simulink model "RL_based_microgrid"  (R2024b)
settings: Solver=VariableStepAuto  StartTime=0.0  StopTime=24  RelTol=1e-3
undefined symbols (not defined in the file): dspblkCoreblockFVToolHelper, gcbh, Ion, Lithium
libraries: spsParallelRLCBranchLib x7, spsSeriesRLCBranchLib x6, spsCurrentMeasurementLib x4, spsPWMGeneratorDCDCLib x4, spsVoltageMeasurementLib x4, spsUniversalBridgeLib x3, spsIGBTDiodeLib x2, spsDiodeLib x2, spsIGBTLib x2, spsBatteryLib x1, spsExcitationSystemLib x1, slpidlib x1
settings Model: Creator=purna  LastModifiedBy=purna

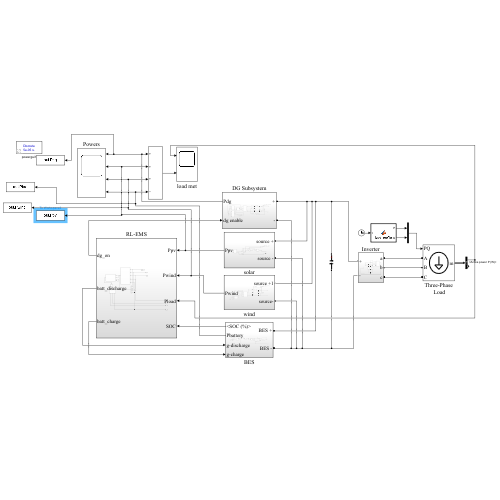
[thumbnail: Simulink's stored preview of the top-level diagram]
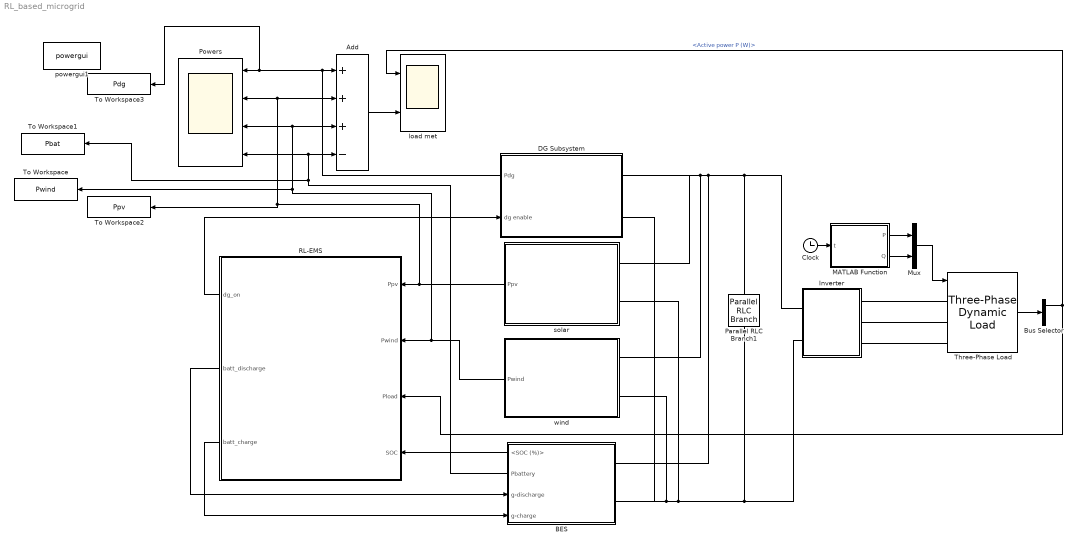
== system RL_based_microgrid ==
  Add : Sum  Inputs=+++-
  BES : Subsystem
      settings: PortSchema="{\"entries\":[{\"content\":{\"sides\":[{\"content\":{\"connectorIds\":[\"Out1\",\"Out2\",\"In1\",\"In2\"]},\"type\":\"ConnectorPlacement.EquallySpacedRectSide\",\"uuid\":\"4ddb1c12-991e-4618-8b5a-96153a6be9f9\"},{\"content\":{\"connectorIds\":[\"RConn1\",\"RConn2\"],\"side\":\"RIGHT\"},\"type\":\"ConnectorPlacement.EquallySpacedRectSide\",\"uuid\":\"57b35f38-742b-43df-b310-85bef7c22eb6\"},{\"content\":{\"side\":\"TOP\"},\"type\":\"ConnectorPlacement.EquallySpacedRectSide\",\"uuid\":\"e8572676-69f6-4b23-a9b1-c7da9405a7b0\"}]},\"type\":\"ConnectorPlacement.EquallySpacedConnector\",\"uuid\":\"66137947-70c4-42b3-9854-4ace8c633b7a\"}],\"packageUris\":[\"http://schema.mathworks.com/mf0/Connector/R2020b\"],\"version\":\"1.0\"}"
  Bus Selector : BusSelector  OutputSignals=Active power P (W),Reactive power Q (var)
  Clock : Clock
  DG Subsystem : Subsystem
      settings: PortSchema="{\"entries\":[{\"content\":{\"sides\":[{\"content\":{\"connectorIds\":[\"LConn1\",\"LConn2\"]},\"type\":\"ConnectorPlacement.EquallySpacedRectSide\",\"uuid\":\"0fe261cd-b61b-4009-ad1d-7ade665678a0\"},{\"content\":{\"connectorIds\":[\"Out1\",\"In1\"],\"side\":\"RIGHT\"},\"type\":\"ConnectorPlacement.EquallySpacedRectSide\",\"uuid\":\"7da4c722-b648-49c7-a33d-9b77a7c6f0e6\"},{\"content\":{\"side\":\"TOP\"},\"type\":\"ConnectorPlacement.EquallySpacedRectSide\",\"uuid\":\"52742111-5208-4731-a6b6-f9628022c544\"}]},\"type\":\"ConnectorPlacement.EquallySpacedConnector\",\"uuid\":\"59f2cf42-9f29-4a8f-af78-3ef44fb976f0\"}],\"packageUris\":[\"http://schema.mathworks.com/mf0/Connector/R2020b\"],\"version\":\"1.0\"}"
  Inverter : Subsystem
  MATLAB Function : MATLAB Function  TreatAsAtomicUnit=on
  Mux : Mux  Inputs=2
  Parallel RLC Branch1 : spsParallelRLCBranchLib/Parallel RLC Branch  LConnTagsString=a  RConnTagsString=__new0  BranchType=C  Resistance=1  Inductance=1e-3  SetiL0=off  InitialCurrent=0  Capacitance=2200e-6  Setx0=off  InitialVoltage=0  Measurements=Branch voltage
  Powers : Scope  NumInputPorts=4
  RL-EMS : Subsystem
  Three-Phase Load : spsThreePhaseDynamicLoadLib/Three-Phase Dynamic Load  NominalVoltage=[ 415 50 ]  ActiveReactivePowers=[12000 5810]  PositiveSequence=[0.994 -11.8]  ExternalControl=on  NpNq=[1.3 2]  TimeConstants="[0  0  0  0]"  MinimumVoltage=0.7  Tfilter=1e-4  LoadFlowParameters=[4,0,0,0,0]
      settings: LibrarySourceBlock=|
      | sps_lib/Passives/Three-Phase
      | Dynamic Load
  To Workspace : ToWorkspace  VariableName=Pwind  SampleTime=-1
  To Workspace1 : ToWorkspace  VariableName=Pbat  SampleTime=-1
  To Workspace2 : ToWorkspace  VariableName=Ppv  SampleTime=-1
  To Workspace3 : ToWorkspace  VariableName=Pdg  SampleTime=-1
  load met : Scope  NumInputPorts=2
  powergui1 : sps_lib/powergui  Priority=1  SimulationMode=Discrete  SampleTime=50e-6  frequency=60  Iterations=50  frequencyindice=0  Pbase=100e6  ErrMax=1e-4  UnitsV=kV  UnitsW=MW  buscounter=0  FunctionMessages=off  echomessages=off  EnableUseOfTLC=off  CurrentSourceSwitches=off  DisableSnubberDevices=off  DisableRonSwitches=off  DisableVfSwitches=off  DisplayEquations=off  AutomaticDiscreteSolvers=off  SolverType=Tustin/Backward Euler (TBE)  Interpol=off  ExternalGateDelay=off  methode=off  Ts=100  x0status=blocks  SPID=on  SwTol=0  HookPort=off  NonlinearTolerance=1e-4  nMaxIteration=100  ContinueOnMaxIteration=off  RestoreLinks=warning  ResistiveCurrentMeasurement=off  Frange=[0:2:500]  Ylog=off  Xlog=on  ShowGrid=off  save=off  variable=ZData  structure=0  ZoomFFT=off  StartTime=0.0  cycles=1  DisplayStyle=1  fundamental=60  FreqAxis=off  MaxFrequency=1000  frequencyindicesteady=1  RmsSteady=1  display=off
  solar : Subsystem
      settings: PortSchema="{\"entries\":[{\"content\":{\"sides\":[{\"content\":{\"connectorIds\":[\"Out1\"]},\"type\":\"ConnectorPlacement.EquallySpacedRectSide\",\"uuid\":\"4201751c-a9df-4880-bfb5-bb337a412f45\"},{\"content\":{\"connectorIds\":[\"RConn1\",\"RConn2\"],\"side\":\"RIGHT\"},\"type\":\"ConnectorPlacement.EquallySpacedRectSide\",\"uuid\":\"9e737d78-7a45-4b12-adbf-ff1ceeb3dd67\"},{\"content\":{\"side\":\"TOP\"},\"type\":\"ConnectorPlacement.EquallySpacedRectSide\",\"uuid\":\"1925966d-444e-49d2-aa13-9b6a49dc85cf\"}]},\"type\":\"ConnectorPlacement.EquallySpacedConnector\",\"uuid\":\"d7480a8d-0b50-46ad-a335-fcb334a83c63\"}],\"packageUris\":[\"http://schema.mathworks.com/mf0/Connector/R2020b\"],\"version\":\"1.0\"}"
  wind : Subsystem
      settings: PortSchema="{\"entries\":[{\"content\":{\"sides\":[{\"content\":{\"connectorIds\":[\"Out1\"]},\"type\":\"ConnectorPlacement.EquallySpacedRectSide\",\"uuid\":\"4201751c-a9df-4880-bfb5-bb337a412f45\"},{\"content\":{\"connectorIds\":[\"RConn1\",\"RConn2\"],\"side\":\"RIGHT\"},\"type\":\"ConnectorPlacement.EquallySpacedRectSide\",\"uuid\":\"9e737d78-7a45-4b12-adbf-ff1ceeb3dd67\"},{\"content\":{\"side\":\"TOP\"},\"type\":\"ConnectorPlacement.EquallySpacedRectSide\",\"uuid\":\"1925966d-444e-49d2-aa13-9b6a49dc85cf\"}]},\"type\":\"ConnectorPlacement.EquallySpacedConnector\",\"uuid\":\"d7480a8d-0b50-46ad-a335-fcb334a83c63\"}],\"packageUris\":[\"http://schema.mathworks.com/mf0/Connector/R2020b\"],\"version\":\"1.0\"}"
  wires:
  Mux/1 -> Three-Phase Load/1
  MATLAB Function/2(Q) -> Mux/2
  Clock/1 -> MATLAB Function/1(t)
  Three-Phase Load/1 -> Bus Selector/1
  MATLAB Function/1(P) -> Mux/1
  RL-EMS/3(batt_charge) -> BES/2(g-charge)
  RL-EMS/2(batt_discharge) -> BES/1(g-discharge)
  RL-EMS/1(dg_on) -> DG Subsystem/1(dg enable)
  solar/1(Ppv) -> Add/2, Powers/2, To Workspace2/1, RL-EMS/1(Ppv)
  wind/1(Pwind) -> RL-EMS/2(Pwind), Add/3, Powers/3, To Workspace/1
  BES/1(<SOC (%)>) -> RL-EMS/4(SOC)
  Bus Selector/1 -> RL-EMS/3(Pload), load met/1  "<Active power P (W)>"
  DG Subsystem/1(Pdg) -> To Workspace3/1, Powers/1, Add/1
  Add/1 -> load met/2
  BES/2(Pbattery) -> Add/4, Powers/4, To Workspace1/1
  connections:
  Inverter/RConn1 -- Parallel RLC Branch1/LConn1 -- BES/RConn1 -- wind/RConn1 -- DG Subsystem/LConn1 -- solar/RConn1
  solar/RConn2 -- wind/RConn2 -- DG Subsystem/LConn2 -- BES/RConn2 -- Parallel RLC Branch1/RConn1 -- Inverter/RConn2
  Three-Phase Load/LConn2 -- Inverter/LConn2
  Three-Phase Load/LConn3 -- Inverter/LConn3
  Three-Phase Load/LConn1 -- Inverter/LConn1

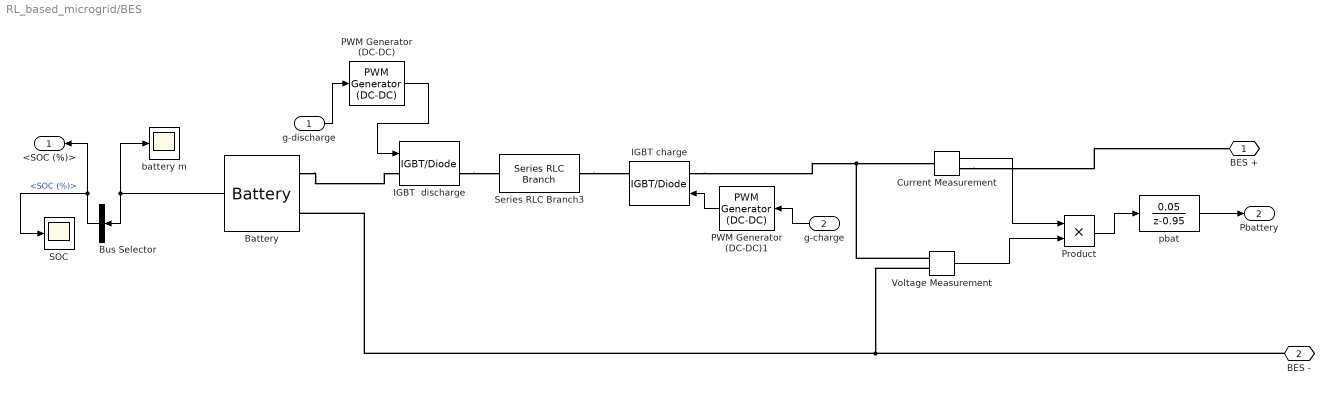
== system RL_based_microgrid/BES ==
  g-discharge : Inport
  g-charge : Inport  Port=2
  Battery : spsBatteryLib/Battery  BatType=Lithium-Ion  NomV=400  NomQ=50  SOC=60  Batt_Tr=0.5  PresetModel=on  MaxQ=50  MinV=300  FullV=465.5949  Dis_rate=21.7391  R=0.08  Normal_OP=45.2174  expZone="[432.1543      2.456522]"
  Bus Selector : BusSelector  OutputSignals=SOC (%)
  Current Measurement : spsCurrentMeasurementLib/Current Measurement  PhasorSimulation=off  OutputType=Complex  PSBequivalent=0
  IGBT  discharge : spsIGBTDiodeLib/IGBT//Diode  Ron=1e-3  Rs=1e5  Cs=inf  Measurements=on
  IGBT charge : spsIGBTDiodeLib/IGBT//Diode  Ron=1e-3  Rs=1e5  Cs=inf  Measurements=on
  PWM Generator (DC-DC) : spsPWMGeneratorDCDCLib/PWM Generator (DC-DC)  Fsw=50000  Ts=1e5
  PWM Generator (DC-DC)1 : spsPWMGeneratorDCDCLib/PWM Generator (DC-DC)  Fsw=50000  Ts=1e5
  Product : Product
  SOC : Scope
  Series RLC Branch3 : spsSeriesRLCBranchLib/Series RLC Branch  LConnTagsString=__new0  RConnTagsString=__new0  BranchType=L  Resistance=1  Inductance=2e-3  SetiL0=off  InitialCurrent=0  Capacitance=1e-6  Setx0=off  InitialVoltage=0  Measurements=None
  Voltage Measurement : spsVoltageMeasurementLib/Voltage Measurement  PhasorSimulation=off  OutputType=Complex  PSBequivalent=0
  battery m : Scope
  pbat : DiscreteTransferFcn  LoadFcn=dspblkCoreblockFVToolHelper(gcbh,'load');  Numerator=[0.05]  Denominator=[1 -0.95]
      settings: CopyFcn=dspblkCoreblockFVToolHelper(gcbh,'copy');  DeleteFcn=dspblkCoreblockFVToolHelper(gcbh,'close');  ModelCloseFcn=dspblkCoreblockFVToolHelper(gcbh,'close');  PreSaveFcn=dspblkCoreblockFVToolHelper(gcbh,'presave');  PostSaveFcn=dspblkCoreblockFVToolHelper(gcbh,'postsave');  CloseFcn=dspblkCoreblockFVToolHelper(gcbh,'close');
  BES + : PMIOPort  Side=Right
  BES - : PMIOPort  Port=2  Side=Right
  <SOC (%)> : Outport
  Pbattery : Outport  Port=2
  wires:
  Bus Selector/1 -> <SOC (%)>/1, SOC/1  "<SOC (%)>"
  Battery/1 -> Bus Selector/1, battery m/1
  g-discharge/1 -> PWM Generator (DC-DC)/1
  PWM Generator (DC-DC)/1 -> IGBT  discharge/1
  PWM Generator (DC-DC)1/1 -> IGBT charge/1
  g-charge/1 -> PWM Generator (DC-DC)1/1
  pbat/1 -> Pbattery/1
  Product/1 -> pbat/1
  Current Measurement/1 -> Product/1
  Voltage Measurement/1 -> Product/2
  connections:
  Series RLC Branch3/RConn1 -- IGBT charge/RConn1
  Battery/LConn1 -- IGBT  discharge/LConn1
  IGBT  discharge/RConn1 -- Series RLC Branch3/LConn1
  BES -/RConn1 -- Voltage Measurement/LConn2 -- Battery/LConn2
  IGBT charge/LConn1 -- Voltage Measurement/LConn1 -- Current Measurement/LConn1
  Current Measurement/RConn1 -- BES +/RConn1

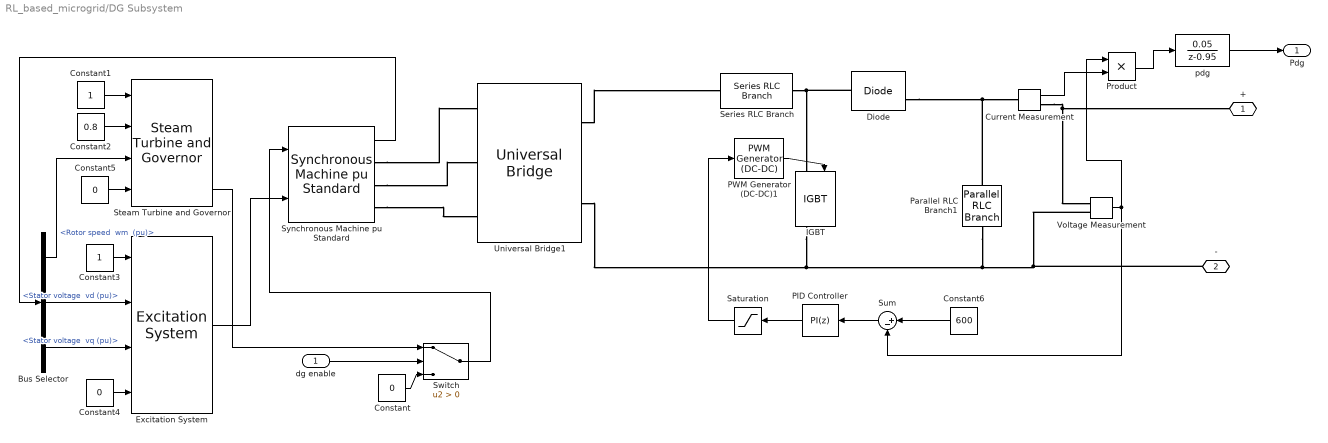
== system RL_based_microgrid/DG Subsystem ==
  dg enable : Inport
  Bus Selector : BusSelector  OutputSignals="Mechanical.Rotor speed  wm  (pu),dq0 components.Stator voltage  vd (pu),dq0 components.Stator voltage  vq (pu)"
  Constant : Constant  Value=0
  Constant1 : Constant
  Constant2 : Constant  Value=0.8
  Constant3 : Constant
  Constant4 : Constant  Value=0
  Constant5 : Constant  Value=0
  Constant6 : Constant  Value=600
  Current Measurement : spsCurrentMeasurementLib/Current Measurement  PhasorSimulation=off  OutputType=Complex  PSBequivalent=0
  Diode : spsDiodeLib/Diode  Ron=0.001  Lon=0  Vf=0.8  IC=0  UseSnubber=0  Rs=500  Cs=0  Measurements=on
  Excitation System : spsExcitationSystemLib/Excitation System  tr=20e-3  reg=[200 0.02]  exc=[ 1, 0.8 ]  tgr=[ 0, 0 ]  damp=[ 0.001, 0.1 ]  sat=[ 0, 0 ]  lim=[-5 5 0]  v0=[1.0 1.0]
  IGBT : spsIGBTLib/IGBT  Ron=0.001  Lon=0  Vf=1  Tf=1e-6  Tt=2e-6  IC=0  Rs=1e5  Cs=inf  Measurements=on
  PID Controller : slpidlib/PID Controller  Controller=PI  Form=Parallel  TimeDomain=Discrete-time  UseExternalTs=off  SampleTime=5e-6  IntegratorMethod=Forward Euler  FilterMethod=Forward Euler  ControllerParametersSource=internal  P=0.002  I=2  UseKiTs=off  D=0  UseExternalDerivativeSource=off  N=100  UseFilter=on  TunerSelectOption=Transfer Function Based (PID Tuner App)  InitialConditionSource=internal  InitialConditionForIntegrator=0  InitialConditionForFilter=0  DifferentiatorICPrevScaledInput=0  ExternalReset=none  TrackingMode=off  Kt=1  LimitOutput=on  SatLimitsSource=internal  UpperSaturationLimit=0.9  LowerSaturationLimit=0  LinearizeAsGain=on  AntiWindupMode=clamping  Kb=1  LimitIntegrator=off  UpperIntegratorSaturationLimit=inf  LowerIntegratorSaturationLimit=-inf  POutMin=[]  POutMax=[]  IOutMin=[]  IOutMax=[]  DOutMin=[]  DOutMax=[]  NOutMin=[]  NOutMax=[]  SumOutMin=[]  SumOutMax=[]  SaturationOutMin=[]  SaturationOutMax=[]  PParamMin=[]  PParamMax=[]  IParamMin=[]  IParamMax=[]  DParamMin=[]  DParamMax=[]  NParamMin=[]  NParamMax=[]  KbParamMin=[]  KbParamMax=[]  KtParamMin=[]  KtParamMax=[]  KbOutMin=[]  KbOutMax=[]  KtOutMin=[]  KtOutMax=[]  IntegratorOutMin=[]  IntegratorOutMax=[]  FilterOutMin=[]  FilterOutMax=[]  SumI1OutMin=[]  SumI1OutMax=[]  SumI2OutMin=[]  SumI2OutMax=[]  SumI3OutMin=[]  SumI3OutMax=[]  SumI4OutMin=[]  SumI4OutMax=[]  SumDOutMin=[]  SumDOutMax=[]  DifferentiatorOutMin=[]  DifferentiatorOutMax=[]  FilterDiffOutCoefMin=[]  FilterDiffOutCoefMax=[]  ReciprocalOutMin=[]  ReciprocalOutMax=[]  SumDenOutMin=[]  SumDenOutMax=[]  SumNumOutMin=[]  SumNumOutMax=[]  DivideOutMin=[]  DivideOutMax=[]  UdiffTsProdOutMin=[]  UdiffTsProdOutMax=[]  NTsProdOutMin=[]  NTsProdOutMax=[]  UintegralTsProdOutMin=[]  UintegralTsProdOutMax=[]  UngainTsProdOutMin=[]  UngainTsProdOutMax=[]  ClampingZeroOutDataTypeStr=Inherit: Inherit via back propagation  ClampingZeroOutMin=[]  ClampingZeroOutMax=[]  FilterDenConstantOutDataTypeStr=Inherit: Inherit via back propagation  FilterDenConstantOutMin=[]  FilterDenConstantOutMax=[]  PCopyOutDataTypeStr=Inherit: Inherit via back propagation  PCopyOutMin=[]  PCopyOutMax=[]  NCopyOutDataTypeStr=Inherit: Inherit via back propagation  NCopyOutMin=[]  NCopyOutMax=[]  IntegratorContinuousStateAttributes=''  IntegratorStateMustResolveToSignalObject=off  IntegratorRTWStateStorageClass=Auto  FilterContinuousStateAttributes=''  FilterStateMustResolveToSignalObject=off  FilterRTWStateStorageClass=Auto  ParallelPVariant=InternalParameters  IdealPVariant=Disabled  IVariant=InternalParameters  DVariant=Disabled  IntegratorVariant=Discrete  SatVariant=Enabled  AWVariant=DiscClampingParallel  PCopyVariant=Disabled  TRVariant=Disabled  FdbkBlocksVariant=Forward  IdealPFdbkVariant=Disabled  SatFdbkVariant=Disabled  DerivativeFilterVariant=Disabled  NVariant=Disabled  NCopyVariant=Disabled_SignalSpec  FilterICVariant=Disabled  IntegratorICVariant=InternalICs  ExternalResetVariant=Disabled  TRSumVariant=Passthrough  SumFdbkVariant=Disabled  SumVariant=Sum_PI  TsampFilterVariant=InternalTs  TsampNgainVariant=Passthrough  TsampIntegralVariant=Disabled_SignalSpec  ExternalSaturationOutDataTypeStr=Inherit: Same as second input  DerivativeSourceVariant=Disabled  PreIntVariant=InternalPreInt
  PWM Generator (DC-DC)1 : spsPWMGeneratorDCDCLib/PWM Generator (DC-DC)  Fsw=10000  Ts=0
  Parallel RLC Branch1 : spsParallelRLCBranchLib/Parallel RLC Branch  LConnTagsString=a  RConnTagsString=__new0  BranchType=C  Resistance=1  Inductance=1e-3  SetiL0=off  InitialCurrent=0  Capacitance=2200e-6  Setx0=off  InitialVoltage=0  Measurements=None
  Product : Product
  Saturation : Saturate  UpperLimit=0.9  LowerLimit=0.02
  Series RLC Branch : spsSeriesRLCBranchLib/Series RLC Branch  LConnTagsString=__new0  RConnTagsString=__new0  BranchType=L  Resistance=1  Inductance=1e-3  SetiL0=off  InitialCurrent=0  Capacitance=1e-6  Setx0=off  InitialVoltage=0  Measurements=None
  Steam Turbine and Governor : spsSteamTurbineandGovernorLib/Steam Turbine and Governor  gentype=Tandem-compound (multi-mass)  reg1="[ 1  0.05    0 ]"  reg2="[ 0.001  0.15 ]"  reg3="[ -0.1  0.1  0  4.496]"  N=3600  turb1="[ 0  10   3.3   0.5   ]"  turb2="[ 0.5   0.5   0  0 ]"  HA="[  1.5498   0.24894  0  0 ]"  KA="[  83.47  42.702  0  0 ]"  DA="[  0.3104  0.05  0  0 ]*8"  ini1=250.35/555  ini2=[2.7247e-008,-120.13]
  Sum : Sum  Inputs=|+-
  Switch : Switch  Criteria=u2 > Threshold  SaturateOnIntegerOverflow=off  InputSameDT=off
  Synchronous Machine pu Standard : spsSynchronousMachinepuStandardLib/Synchronous Machine pu Standard  PresetModel=No  MechanicalLoad=Mechanical power Pm  ShowDetailedParameters=on  RotorType=Salient-pole  Units=per unit standard parameters  MeasurementBus=off  NominalParameters="[ 50e3   415   50   2 ]"  Reactances1=[ 1.81, 0.3, 0.23, 1.76, 0.65, 0.25, 0.15 ]  Reactances2=[2.24 0.17 0.12 1.02 0.13 0.08]  dAxisTimeConstants=Short-circuit  qAxisTimeConstants=Short-circuit  TimeConstants1="[ 4.4849  0.0681  0.1  ]"  TimeConstants2=[ 8.0, 0.03, 1.0, 0.07 ]  TimeConstants3="[  4.49  0.0681  0.0513  ]"  TimeConstants4=[ 8.0, 0.03, 0.3371, 0.0295 ]  TimeConstants5=[ 1.01, 0.053, 0.1 ]  TimeConstants6=[ 1.3201, 0.023, 1.0, 0.07 ]  TimeConstants7=[0.012 0.003 0.003]  TimeConstants8=[ 1.3201, 0.0231, 0.3371, 0.0295 ]  StatorResistance=0.037875  Mechanical=[0.1028 0.02056 2]  PolePairs=20  InitialConditions="[ 0  0  0  0  0  0  0  0  1 ]"  SetSaturation=off  Saturation=[0.6404,0.7127,0.8441,0.9214,0.9956,1.082,1.19,1.316,1.457;0.7,0.7698,0.8872,0.9466,0.9969,1.046,1.1,1.151,1.201]  LoadFlowParameters=[1,0,0,0,0]  TsPowergui=0  TsBlock=5e-05  IterativeModel=Trapezoidal non iterative  IterativeDiscreteModel=Trapezoidal non iterative  BusType=swing  Pref=20000  Qref=0  Qmin=-15000  Qmax=15000  PLF=0  QLF=0
  Universal Bridge1 : spsUniversalBridgeLib/Universal Bridge  Arms=3  SnubberResistance=1e5  SnubberCapacitance=inf  Device=Diodes  Ron=1e-3  Lon=0  ForwardVoltages="[  0  0  ]"  ForwardVoltage=0  GTOparameters=[ 10e-6 , 20e-6 ]  IGBTparameters=[ 1e-6 , 2e-6 ]  Measurements=None  Measurements_2=None  converterType=Rectifier
  Voltage Measurement : spsVoltageMeasurementLib/Voltage Measurement  PhasorSimulation=off  OutputType=Complex  PSBequivalent=0
  pdg : DiscreteTransferFcn  LoadFcn=dspblkCoreblockFVToolHelper(gcbh,'load');  Numerator=[0.05]  Denominator=[1 -0.95]
      settings: CopyFcn=dspblkCoreblockFVToolHelper(gcbh,'copy');  DeleteFcn=dspblkCoreblockFVToolHelper(gcbh,'close');  ModelCloseFcn=dspblkCoreblockFVToolHelper(gcbh,'close');  PreSaveFcn=dspblkCoreblockFVToolHelper(gcbh,'presave');  PostSaveFcn=dspblkCoreblockFVToolHelper(gcbh,'postsave');  CloseFcn=dspblkCoreblockFVToolHelper(gcbh,'close');
  + : PMIOPort  Side=Left
  - : PMIOPort  Port=2  Side=Left
  Pdg : Outport
  wires:
  Constant3/1 -> Excitation System/1
  Bus Selector/3 -> Excitation System/3  "<Stator voltage  vq (pu)>"
  Constant4/1 -> Excitation System/4
  Bus Selector/1 -> Steam Turbine and Governor/3  "<Rotor speed  wm  (pu)>"
  Constant2/1 -> Steam Turbine and Governor/2
  Bus Selector/2 -> Excitation System/2  "<Stator voltage  vd (pu)>"
  Constant1/1 -> Steam Turbine and Governor/1
  Constant5/1 -> Steam Turbine and Governor/4
  Excitation System/1 -> Synchronous Machine pu Standard/2
  Synchronous Machine pu Standard/1 -> Bus Selector/1
  Constant/1 -> Switch/3
  dg enable/1 -> Switch/2
  Product/1 -> pdg/1
  Current Measurement/1 -> Product/2
  pdg/1 -> Pdg/1
  Steam Turbine and Governor/4 -> Switch/1
  Switch/1 -> Synchronous Machine pu Standard/1
  PWM Generator (DC-DC)1/1 -> IGBT/1
  Voltage Measurement/1 -> Sum/2, Product/1
  Sum/1 -> PID Controller/1
  Saturation/1 -> PWM Generator (DC-DC)1/1
  PID Controller/1 -> Saturation/1
  Constant6/1 -> Sum/1
  connections:
  Synchronous Machine pu Standard/RConn3 -- Universal Bridge1/LConn3
  Synchronous Machine pu Standard/RConn1 -- Universal Bridge1/LConn1
  Synchronous Machine pu Standard/RConn2 -- Universal Bridge1/LConn2
  Parallel RLC Branch1/LConn1 -- Diode/RConn1 -- Current Measurement/LConn1
  IGBT/RConn1 -- Universal Bridge1/RConn2 -- Parallel RLC Branch1/RConn1 -- Voltage Measurement/LConn2 -- -/RConn1
  Current Measurement/RConn1 -- +/RConn1 -- Voltage Measurement/LConn1
  Series RLC Branch/RConn1 -- Diode/LConn1 -- IGBT/LConn1
  Universal Bridge1/RConn1 -- Series RLC Branch/LConn1

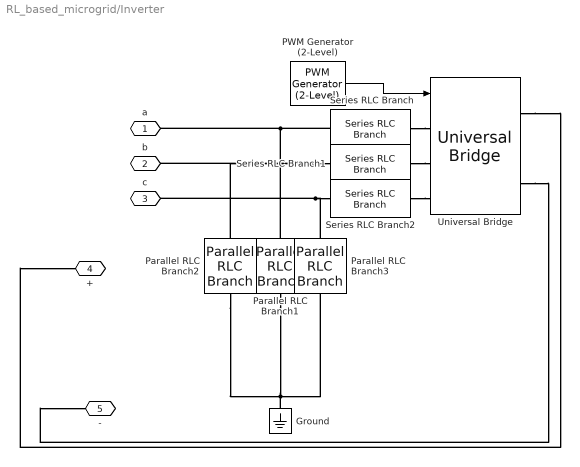
== system RL_based_microgrid/Inverter ==
  Ground : spsGroundLib/Ground  LConnTagsString=a
  PWM Generator (2-Level) : spsPWMGenerator2LevelLib/PWM Generator (2-Level)  ModulatorType=Three-phase bridge (6 pulses)  ModulatorMode=Unsynchronized  Fc=5000  Pc=0  nF=27  MinMax="[ -1  1 ]"  SamplingTechnique=Natural  ModulatingSignals=on  m=0.8  Freq=50  Phase=0  Ts=0  ShowCarrierOutport=off
  Parallel RLC Branch1 : spsParallelRLCBranchLib/Parallel RLC Branch  LConnTagsString=a  RConnTagsString=__new0  BranchType=C  Resistance=1  Inductance=1e-3  SetiL0=off  InitialCurrent=0  Capacitance=20e-6  Setx0=off  InitialVoltage=0  Measurements=None
  Parallel RLC Branch2 : spsParallelRLCBranchLib/Parallel RLC Branch  LConnTagsString=a  RConnTagsString=__new0  BranchType=C  Resistance=1  Inductance=1e-3  SetiL0=off  InitialCurrent=0  Capacitance=20e-6  Setx0=off  InitialVoltage=0  Measurements=None
  Parallel RLC Branch3 : spsParallelRLCBranchLib/Parallel RLC Branch  LConnTagsString=a  RConnTagsString=__new0  BranchType=C  Resistance=1  Inductance=1e-3  SetiL0=off  InitialCurrent=0  Capacitance=20e-6  Setx0=off  InitialVoltage=0  Measurements=None
  Series RLC Branch : spsSeriesRLCBranchLib/Series RLC Branch  LConnTagsString=__new0  RConnTagsString=__new0  BranchType=L  Resistance=1  Inductance=2e-3  SetiL0=off  InitialCurrent=0  Capacitance=1e-6  Setx0=off  InitialVoltage=0  Measurements=None
  Series RLC Branch1 : spsSeriesRLCBranchLib/Series RLC Branch  LConnTagsString=__new0  RConnTagsString=__new0  BranchType=L  Resistance=1  Inductance=2e-3  SetiL0=off  InitialCurrent=0  Capacitance=1e-6  Setx0=off  InitialVoltage=0  Measurements=None
  Series RLC Branch2 : spsSeriesRLCBranchLib/Series RLC Branch  LConnTagsString=__new0  RConnTagsString=__new0  BranchType=L  Resistance=1  Inductance=2e-3  SetiL0=off  InitialCurrent=0  Capacitance=1e-6  Setx0=off  InitialVoltage=0  Measurements=None
  Universal Bridge : spsUniversalBridgeLib/Universal Bridge  Arms=3  SnubberResistance=1e5  SnubberCapacitance=inf  Device=IGBT / Diodes  Ron=1e-3  Lon=0  ForwardVoltages="[  0  0  ]"  ForwardVoltage=0  GTOparameters=[ 10e-6 , 20e-6 ]  IGBTparameters=[ 1e-6 , 2e-6 ]  Measurements=None  Measurements_2=None  converterType=Rectifier
  a : PMIOPort  Side=Left
  b : PMIOPort  Port=2  Side=Left
  c : PMIOPort  Port=3  Side=Left
  + : PMIOPort  Port=4  Side=Right
  - : PMIOPort  Port=5  Side=Right
  wires:
  PWM Generator (2-Level)/1 -> Universal Bridge/1
  connections:
  Parallel RLC Branch2/RConn1 -- Ground/LConn1 -- Parallel RLC Branch1/RConn1 -- Parallel RLC Branch3/RConn1
  Series RLC Branch/RConn1 -- Universal Bridge/LConn1
  Series RLC Branch1/RConn1 -- Universal Bridge/LConn2
  Series RLC Branch2/RConn1 -- Universal Bridge/LConn3
  Universal Bridge/RConn2 -- -/RConn1
  Parallel RLC Branch3/LConn1 -- c/RConn1 -- Series RLC Branch2/LConn1
  Series RLC Branch/LConn1 -- Parallel RLC Branch1/LConn1 -- a/RConn1
  Universal Bridge/RConn1 -- +/RConn1
  Series RLC Branch1/LConn1 -- b/RConn1 -- Parallel RLC Branch2/LConn1

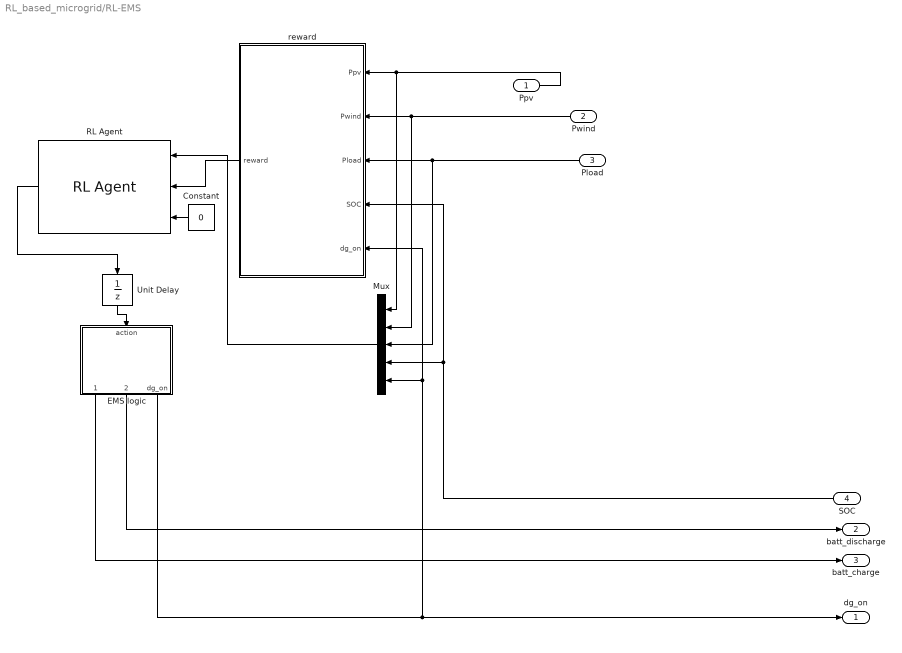
== system RL_based_microgrid/RL-EMS ==
  Ppv : Inport
  Pwind : Inport  Port=2
  Pload : Inport  Port=3
  SOC : Inport  Port=4
  Constant : Constant  Value=0
  EMS logic : MATLAB Function  TreatAsAtomicUnit=on
  Mux : Mux  Inputs=5
  RL Agent : rllib/RL Agent  Agent=agentObj  ExternalActionAsInput=off  ProvideLastAction=off  ProvideCumRwd=off  TreatAsDirectFeedthrough=on  UseStrictObservationDataTypes=off
  Unit Delay : UnitDelay  InitialCondition=2  SampleTime=-1  HasFrameUpgradeWarning=on
  reward : MATLAB Function  TreatAsAtomicUnit=on
  dg_on : Outport
  batt_discharge : Outport  Port=2
  batt_charge : Outport  Port=3
  wires:
  Constant/1 -> RL Agent/3
  SOC/1 -> reward/4(SOC), Mux/4
  Pload/1 -> Mux/3, reward/3(Pload)
  EMS logic/3(dg_on) -> dg_on/1, reward/5(dg_on), Mux/5
  Pwind/1 -> Mux/2, reward/2(Pwind)
  Ppv/1 -> Mux/1, reward/1(Ppv)
  Mux/1 -> RL Agent/1
  RL Agent/1 -> Unit Delay/1
  reward/1(reward) -> RL Agent/2
  EMS logic/1(batt_charge) -> batt_charge/1
  EMS logic/2(batt_discharge) -> batt_discharge/1
  Unit Delay/1 -> EMS logic/1(action)

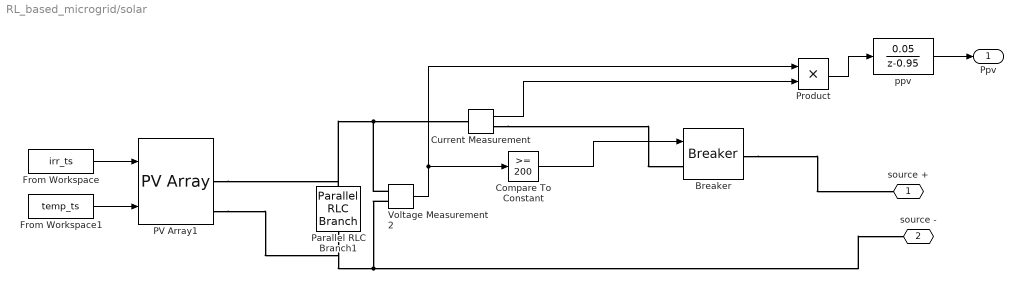
== system RL_based_microgrid/solar ==
  Breaker : spsBreakerLib/Breaker  InitialState=0  SwitchingTimes="[1/60  5/60]"  External=on  BreakerResistance=0.01  SnubberResistance=1e6  SnubberCapacitance=inf  Measurements=None  MoreParameters=on  NoBreakLoop=off
  Compare To Constant : simulink/Logic and Bit Operations/Compare To Constant  relop=>=  const=200  OutDataTypeStr=boolean
  Current Measurement : spsCurrentMeasurementLib/Current Measurement  PhasorSimulation=off  OutputType=Complex  PSBequivalent=0
  From Workspace : FromWorkspace  VariableName=irr_ts  SampleTime=0.01
  From Workspace1 : FromWorkspace  VariableName=temp_ts  SampleTime=0.01
  PV Array1 : spsPVArrayLib/PV Array  Npar=4  Nser=20  PlotType=array @ 1000 W/m2 & specified temperatures  S_vec="[ 1000  500  100 ]"  Temp_C_vec="[ 25 45  ]"  ModuleName=User-defined  PlotWhenSelected=off  Pm=324  Ncell=60  Voc=45  Isc=9.2  Vm=36  Im=9  beta_Voc_pc=-0.36099  alpha_Isc_pc=0.102  beta_Voc=-0.16245  alpha_Isc=0.009384  IL=9.4197  I0=3.4412e-10  nI=1.2147  Rsh=3652.5591  Rs=0.39728  RobustModel=off  RobustCellTemperature=313.3991  BAL=on  Tc=1e-6  Tfilter=5e-5
  Parallel RLC Branch1 : spsParallelRLCBranchLib/Parallel RLC Branch  LConnTagsString=a  RConnTagsString=__new0  BranchType=C  Resistance=1  Inductance=1e-3  SetiL0=off  InitialCurrent=0  Capacitance=2200e-6  Setx0=off  InitialVoltage=0  Measurements=None
  Product : Product
  Voltage Measurement2 : spsVoltageMeasurementLib/Voltage Measurement  PhasorSimulation=off  OutputType=Complex  PSBequivalent=0
  ppv : DiscreteTransferFcn  LoadFcn=dspblkCoreblockFVToolHelper(gcbh,'load');  Numerator=[0.05]  Denominator=[1 -0.95]
      settings: CopyFcn=dspblkCoreblockFVToolHelper(gcbh,'copy');  DeleteFcn=dspblkCoreblockFVToolHelper(gcbh,'close');  ModelCloseFcn=dspblkCoreblockFVToolHelper(gcbh,'close');  PreSaveFcn=dspblkCoreblockFVToolHelper(gcbh,'presave');  PostSaveFcn=dspblkCoreblockFVToolHelper(gcbh,'postsave');  CloseFcn=dspblkCoreblockFVToolHelper(gcbh,'close');
  source + : PMIOPort  Side=Right
  source - : PMIOPort  Port=2  Side=Right
  Ppv : Outport
  wires:
  From Workspace/1 -> PV Array1/1
  From Workspace1/1 -> PV Array1/2
  Current Measurement/1 -> Product/2
  Product/1 -> ppv/1
  Voltage Measurement2/1 -> Product/1, Compare To Constant/1
  ppv/1 -> Ppv/1
  Compare To Constant/1 -> Breaker/1
  connections:
  Voltage Measurement2/LConn1 -- PV Array1/RConn1 -- Parallel RLC Branch1/LConn1 -- Current Measurement/LConn1
  Voltage Measurement2/LConn2 -- Parallel RLC Branch1/RConn1 -- PV Array1/RConn2 -- source -/RConn1
  Current Measurement/RConn1 -- Breaker/LConn1
  Breaker/RConn1 -- source +/RConn1

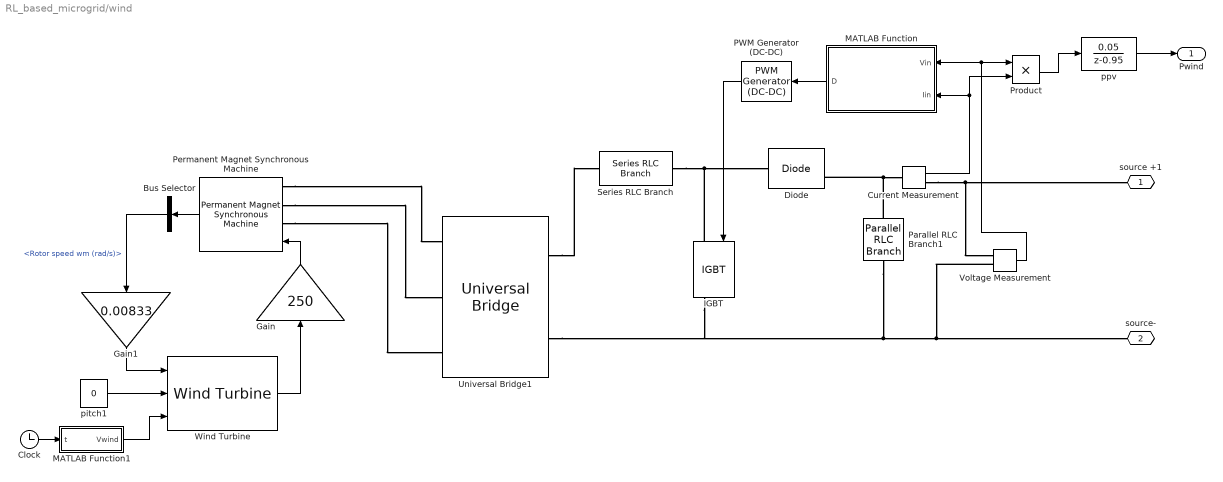
== system RL_based_microgrid/wind ==
  Bus Selector : BusSelector  OutputSignals=Rotor speed wm (rad/s)
  Clock : Clock
  Current Measurement : spsCurrentMeasurementLib/Current Measurement  PhasorSimulation=off  OutputType=Complex  PSBequivalent=0
  Diode : spsDiodeLib/Diode  Ron=0.001  Lon=0  Vf=0.8  IC=0  UseSnubber=0  Rs=500  Cs=0  Measurements=on
  Gain : Gain  Gain=250
  Gain1 : Gain  Gain=0.00833
  IGBT : spsIGBTLib/IGBT  Ron=0.001  Lon=0  Vf=1  Tf=1e-6  Tt=2e-6  IC=0  Rs=1e5  Cs=inf  Measurements=on
  MATLAB Function : MATLAB Function  TreatAsAtomicUnit=on
  MATLAB Function1 : MATLAB Function  TreatAsAtomicUnit=on
  PWM Generator (DC-DC) : spsPWMGeneratorDCDCLib/PWM Generator (DC-DC)  Fsw=10000  Ts=0
  Parallel RLC Branch1 : spsParallelRLCBranchLib/Parallel RLC Branch  LConnTagsString=a  RConnTagsString=__new0  BranchType=C  Resistance=1  Inductance=1e-3  SetiL0=off  InitialCurrent=0  Capacitance=1100e-6  Setx0=off  InitialVoltage=0  Measurements=Branch voltage
  Permanent Magnet Synchronous Machine : spsPermanentMagnetSynchronousMachineLib/Permanent Magnet Synchronous Machine  NbPhases=3  FluxDistribution=Sinusoidal  RotorType=Round  MechanicalLoad=Torque Tm  PresetModel=No  ShowDetailedParameters=on  MeasurementBus=off  Resistance=0.425  Inductance=8.5e-3  dqInductances=[8.5e-3,8.5e-3]  La=0.0085  MachineConstant=Flux linkage established by magnets (V.s)  Flux=0.433  VoltageCst=314.15  TorqueCst=2.598  Flat=120  Mechanical=[0.02 0.001 4 0]  PolePairs=4  InitialConditions=[0,0, 0,0]  InitialConditions5ph=[0 0 0 0 0 0]  RefAngle=90 degrees behind phase A axis (modified Park)  IterativeDiscreteModel=Trapezoidal non iterative  TsBlock=-1  TsPowergui=0
  Product : Product
  Series RLC Branch : spsSeriesRLCBranchLib/Series RLC Branch  LConnTagsString=__new0  RConnTagsString=__new0  BranchType=L  Resistance=1  Inductance=1e-3  SetiL0=off  InitialCurrent=0  Capacitance=1e-6  Setx0=off  InitialVoltage=0  Measurements=None
  Universal Bridge1 : spsUniversalBridgeLib/Universal Bridge  Arms=3  SnubberResistance=1e5  SnubberCapacitance=inf  Device=Diodes  Ron=1e-3  Lon=0  ForwardVoltages="[  0  0  ]"  ForwardVoltage=0  GTOparameters=[ 10e-6 , 20e-6 ]  IGBTparameters=[ 1e-6 , 2e-6 ]  Measurements=None  Measurements_2=None  converterType=Rectifier
  Voltage Measurement : spsVoltageMeasurementLib/Voltage Measurement  PhasorSimulation=off  OutputType=Complex  PSBequivalent=0
  Wind Turbine : spsWindTurbineLib/Wind Turbine  Pnom=30e3  Pelec_base=30e3/0.9  wind_base=12  P_wind_base=1  speed_nom=1  pitch_angle=0  c1_c6="[0.51763          116          0.4            5           21     0.006795]"  cp_nom=0.48  lambda_nom=8.1
  pitch1 : Constant  Value=0
  ppv : DiscreteTransferFcn  LoadFcn=dspblkCoreblockFVToolHelper(gcbh,'load');  Numerator=[0.05]  Denominator=[1 -0.95]
      settings: CopyFcn=dspblkCoreblockFVToolHelper(gcbh,'copy');  DeleteFcn=dspblkCoreblockFVToolHelper(gcbh,'close');  ModelCloseFcn=dspblkCoreblockFVToolHelper(gcbh,'close');  PreSaveFcn=dspblkCoreblockFVToolHelper(gcbh,'presave');  PostSaveFcn=dspblkCoreblockFVToolHelper(gcbh,'postsave');  CloseFcn=dspblkCoreblockFVToolHelper(gcbh,'close');
  source +1 : PMIOPort  Side=Right
  source- : PMIOPort  Port=2  Side=Right
  Pwind : Outport
  wires:
  pitch1/1 -> Wind Turbine/2
  Permanent Magnet Synchronous Machine/1 -> Bus Selector/1
  Product/1 -> ppv/1
  Current Measurement/1 -> Product/2, MATLAB Function/2(Iin)
  ppv/1 -> Pwind/1
  Voltage Measurement/1 -> Product/1, MATLAB Function/1(Vin)
  Gain/1 -> Permanent Magnet Synchronous Machine/1
  Bus Selector/1 -> Gain1/1  "<Rotor speed wm (rad/s)>"
  Gain1/1 -> Wind Turbine/1
  Wind Turbine/1 -> Gain/1
  MATLAB Function/1(D) -> PWM Generator (DC-DC)/1
  PWM Generator (DC-DC)/1 -> IGBT/1
  Clock/1 -> MATLAB Function1/1(t)
  MATLAB Function1/1(Vwind) -> Wind Turbine/3
  connections:
  Permanent Magnet Synchronous Machine/LConn1 -- Universal Bridge1/LConn3
  Permanent Magnet Synchronous Machine/LConn2 -- Universal Bridge1/LConn2
  Permanent Magnet Synchronous Machine/LConn3 -- Universal Bridge1/LConn1
  Parallel RLC Branch1/RConn1 -- Voltage Measurement/LConn2 -- source-/RConn1 -- IGBT/RConn1 -- Universal Bridge1/RConn2
  Current Measurement/RConn1 -- Voltage Measurement/LConn1 -- source +1/RConn1
  Parallel RLC Branch1/LConn1 -- Diode/RConn1 -- Current Measurement/LConn1
  Universal Bridge1/RConn1 -- Series RLC Branch/LConn1
  Series RLC Branch/RConn1 -- IGBT/LConn1 -- Diode/LConn1

== matlab function RL_based_microgrid/wind/MATLAB Function ==
  data: Vin input; D output; Iin input
function D = wind_mppt(Vin, Iin)
% wind_mppt
% P&O based MPPT for wind energy system
%
% Inputs:
% Vin - rectifier output voltage (V)
% Iin - rectifier output current (A)
%
% Output:
% D   - duty cycle for boost converter (0 to 0.95)

persistent P_prev V_prev D_prev

if isempty(P_prev)
    P_prev = 0;
    V_prev = 0;
    D_prev = 0.5;   % initial duty cycle
end

% Present power
P = Vin * Iin;

% Step size
step = 0.002;

% P&O logic
if P > P_prev
    if Vin > V_prev
        D = D_prev + step;
    else
        D = D_prev - step;
    end
else
    if Vin > V_prev
        D = D_prev - step;
    else
        D = D_prev + step;
    end
end

% Limit duty cycle
if D > 0.95
    D = 0.95;
elseif D < 0.05
    D = 0.05;
end

% Store previous values
P_prev = P;
V_prev = Vin;
D_prev = D;
end

== matlab function RL_based_microgrid/MATLAB Function ==
  data: t input; P output; Q output
function [P, Q] = load_profile(t)

pf = 0.9;
phi = acos(pf);

if t >= 0 && t < 5
    P = 12e3;
elseif t >= 5 && t < 8
    P = (12 + (t-5)*(18/3))*1e3;
elseif t >= 8 && t < 12
    P = (28 + 2*sin((t-8)*pi/4))*1e3;
elseif t >= 12 && t < 17
    P = (30 + 5*sin((t-12)*pi/5))*1e3;
elseif t >= 17 && t < 22
    P = (35 + 15*sin((t-17)*pi/5))*1e3;
else
    P = 20e3;
end

Q = P * tan(phi);
end

== matlab function RL_based_microgrid/wind/MATLAB Function1 ==
  data: t input; Vwind output
function Vwind = wind_profile(t)
% wind_profile
% 24-hour wind speed variation profile
% (Simulation: 1 sec = 1 hour)

if t >= 0 && t < 4
    Vwind = 4;   % low wind (night)

elseif t >= 4 && t < 8
    Vwind = 6;   % moderate wind (early morning)

elseif t >= 8 && t < 12
    Vwind = 9;   % increasing wind (morning)

elseif t >= 12 && t < 16
    Vwind = 11;  % peak wind (afternoon)

elseif t >= 16 && t < 20
    Vwind = 8;   % decreasing wind (evening)

else
    Vwind = 5;   % low wind (late night)
end

end

== matlab function RL_based_microgrid/RL-EMS/reward ==
  data: Ppv input; reward output; Pwind input; Pload input; SOC input; dg_on input
function reward = rewardFcn(Ppv,Pwind,Pload,SOC,dg_on)

renewable = Ppv + Pwind;

reward = 0;

reward = reward - 10*dg_on;

reward = reward + 0.05*renewable;

if SOC < 30 || SOC > 90
    reward = reward - 5;
end

power_error = abs(Pload - renewable);

reward = reward - 0.02*power_error;

== matlab function RL_based_microgrid/RL-EMS/EMS logic ==
  data: action input; batt_charge output; batt_discharge output; dg_on output
function [batt_charge, batt_discharge, dg_on] = EMS_logic(action)

% Initialize outputs
batt_charge = 0;
batt_discharge = 0;
dg_on = 0;

% RL action decoding
if action == 1
    
    batt_charge = 1;
    batt_discharge = 0;
    dg_on = 0;

elseif action == 2
    
    batt_charge = 0;
    batt_discharge = 0;
    dg_on = 0;

elseif action == 3
    
    batt_charge = 0;
    batt_discharge = 1;
    dg_on = 0;

elseif action == 4
    
    batt_charge = 0;
    batt_discharge = 0;
    dg_on = 1;

end
